simulink model "Counter"  (R2023a)
settings: Solver=VariableStepAuto  StartTime=0.0  StopTime=10.0  RelTol=1e-3
settings Model: Creator=ADMIN  LastModifiedBy=ADMIN

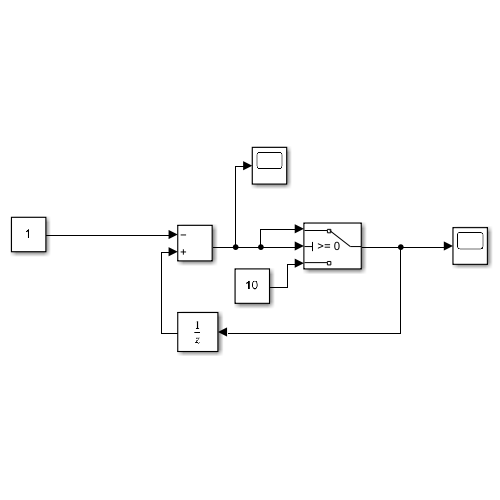
[thumbnail: Simulink's stored preview of the top-level diagram]
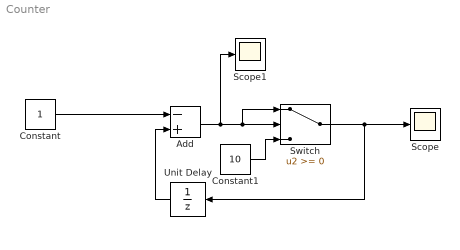
== system Counter ==
  Add : Sum  Inputs=-+
  Constant : Constant
  Constant1 : Constant  Value=10
  Scope : Scope
  Scope1 : Scope
  Switch : Switch  SaturateOnIntegerOverflow=off  InputSameDT=off
  Unit Delay : UnitDelay  SampleTime=-1  HasFrameUpgradeWarning=on
  wires:
  Constant/1 -> Add/1
  Unit Delay/1 -> Add/2
  Add/1 -> Scope1/1, Switch/1, Switch/2
  Switch/1 -> Unit Delay/1, Scope/1
  Constant1/1 -> Switch/3
